simulink model "Communication_Testing"  (R2024a)
settings: Solver=FixedStepAuto  StartTime=0.0  StopTime=100  RelTol=1e-3  EnableMultiTasking=on
undefined symbols (not defined in the file or in its folder): CAN, FD
libraries: stmutilitieslib x29, simulink x25, stm32blockslib x11, canfdmsglib x7, stm32h7xxblockslib x3, dspstat3 x3, slpidlib x2
(part 1 of 2)
settings Model: STM32="{\"FDCANWrite\":[{\"ID\":\"Communication_Testing:678\"},{\"ID\":\"Communication_Testing:677\"},{\"ID\":\"Communication_Testing:1794\"},{\"ID\":\"Communication_Testing:617\"},{\"ID\":\"Communication_Testing:630\"},{\"ID\":\"Communication_Testing:2155\"},{\"ID\":\"Communication_Testing:2156\"}],\"HardwareInterrupt\":[{\"ID\":\"Communication_Testing:1261\"},{\"ID\":\"Communication_Testing:278\"}],\"FDCANRead\":{\"ID\":\"Communication_Testing:282\"},\"AnalogInputForH7\":{\"ID\":\"Communication_Testing:1796\"}}"  Creator=ezeki  LastModifiedBy=ezeki
settings SolverCC: PositivePriorityOrder=on  AutoInsertRateTranBlk=on
settings OptimizationCC: DefaultParameterBehavior=Inlined  EnhancedBackFolding=on  PassReuseOutputArgsAs=Individual arguments  ZeroExternalMemoryAtStartup=off  ZeroInternalMemoryAtStartup=off  MaxStackSize=512  OptimizeBlockOrder=speed  DifferentSizesBufferReuse=on  OptimizationCustomize=off  EfficientTunableParamExpr=on
settings DebuggingCC: ParameterTunabilityLossMsg=error
settings HardwareCC: ProdBitPerPointer=32  ProdBitPerSizeT=32  ProdBitPerPtrDiffT=32  ProdLargestAtomicInteger=Long  ProdLargestAtomicFloat=Double  ProdWordSize=32  ProdLongLongMode=on  ProdHWDeviceType=ARM Compatible->ARM Cortex-M
settings SFSimCC: MATLABDynamicMemAlloc=off
settings RTWCC: Description=Embedded Coder  SystemTargetFile=ert.tlc  HardwareBoard=STM32H7xx Based (Single-core)  TLCOptions="-aInlineSetEventsForThisBaseRateFcn=TLC_FALSE -aSuppressMultiTaskScheduler=TLC_FALSE  -aRateBasedStepFcn=0"  TemplateMakefile=ert_default_tmf  Toolchain=GNU Tools for ARM Embedded Processors  BuildConfiguration=Faster Runs
settings CodeAppCC: ForceParamTrailComments=on  IgnoreCustomStorageClasses=off  OperatorAnnotations=on  SimulinkDataObjDesc=on  SFDataObjDesc=on  InsertBlockDesc=on
settings ERTTargetCC: TargetLangStandard=C99 (ISO)  CodeReplacementLibrary=ARM Cortex-M  ExtModeTransport=3  ExtModeStaticAlloc=on  ExtModeStaticAllocSize=2048  ExtModeMexFile=ext_xcp  ExtModeIntrfLevel=Level2 - Open

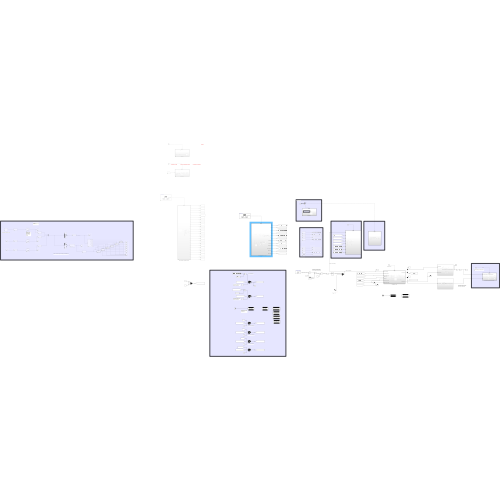
[thumbnail: Simulink's stored preview of the top-level diagram]
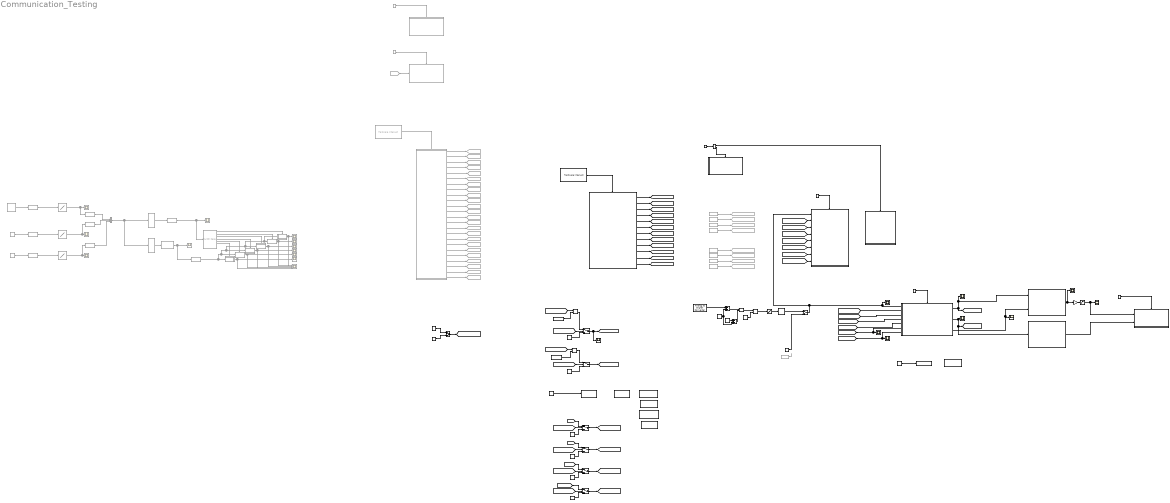
== system Communication_Testing ==
  note: Output to Control Model
  note: Output to CAN for visibility
  note: This invert is done as the right motor spins clockwise. compared to the left motor which spins anticlockwise.
  note: Pot turned down all the way wasnt quite showing 0, this offset was added to ensure 0 throttle could be acheived.
  note: maps 0-3.3V to 0 - 65,536
  note: Traction Control
  note: For testing purposes only
  note: CAN 2 Receive Data From Inverters
  note: Forwarding Messages From the Inverters to Data Logger
  note: This was made for testing the unmultiplexing of Inverter Messages
  note: Inverter Can Setup
  note: A look up table of CAN ID's which are used to request cyclic transmission of data from the inverters
  note: Counter Selects which ID to send
  note: Byte 0 tells the inverters you are setting up cyclic messaging.
  note: CAN 1 information from pedal box and dash.
  note: Set to 500 Hz call
  note: This Constant Can be changed to varible at a latter date for data playback/simulation
  note: Less then 90 enables regen
  note: Greater then 5 enables regen
  note: Greater then 5 enables regen
  note: Converts RPM to Rad/s
  note: This Constant Can be changed to varible at a latter date for data playback/simulation
  note: Example On How to send Messages to Inverters
  note: PID Loop runs allot faster to minimise overshoot. Messages are sent at a slower rate.
  note: Handy to test Can outputs. A constant can be put in to test transmission
  1-D Lookup Table : Lookup_n-D  Commented=on  NumberOfTableDimensions=1  BreakpointsForDimension1=[0 1 2 3 4 5]  Table=[235 74 168 73 95 138]  InterpMethod=Nearest  InternalRulePriority=Speed  RndMeth=Simplest
  1-D Lookup Table1 : Lookup_n-D  Commented=on  NumberOfTableDimensions=1  BreakpointsForDimension1=[0 1 2 3 4 5]  Table=[25 200 25 200 50 50]  InterpMethod=Nearest  InternalRulePriority=Speed  RndMeth=Simplest
  1-D Lookup Table2 : Lookup_n-D  Commented=on  NumberOfTableDimensions=1  BreakpointsForDimension1=[0 1 2 3 4 5]  Table=[25 200 25 200 50 50]  InterpMethod=Nearest  InternalRulePriority=Speed  RndMeth=Simplest
  10 HZ Send : Subsystem  Commented=on  TreatAsAtomicUnit=on
  10 HZ Send1 : Subsystem  TreatAsAtomicUnit=on
  50 HZ Send Torque Requests to Inverters1 : Subsystem  TreatAsAtomicUnit=on
  50 HZ Send1 : Subsystem  Commented=on  TreatAsAtomicUnit=on
  Add : Sum
  Add1 : Sum
  Analog to Digital Converter : stm32h7xxblockslib/Analog to Digital Converter  ADCModule=ADC1  ConversionGroup=Regular  TriggerMode=Trigger and read  NumberOfConversions=1  EnableBufferConv=off  BufferLength=1  OutputStatus=off  SampleTime=-1  EnableSimPort=off  hoistedMaskSrc=ECSoC/ECSimCodegen/Analog to Digital Converter
  Byte Unpack1 : stmutilitieslib/Byte Unpack  Commented=on  dimensions={[1]}  datatypes={'uint16'}  byteAlign=1  blockPlatform=stm32f4discovery
  Constant{,1..3,5..6,10} (7 alike) : Constant  Commented=on  Value=0
  Constant11 : Constant  Commented=on  Value=25000
  Constant12 : Constant  Value=100
  Constant13 : Constant  Value=10000
  Constant14 : Constant  Value=100
  Constant15 : Constant  Value=100
  Constant16 : Constant  Value=0.10472
  Constant17 : Constant  Value=0.10472
  Constant18 : Constant  Value=50
  Constant19 : Constant  Value=85
  Constant20 : Constant  Value=50
  Constant21 : Constant  Value=20
  Constant22 : Constant
  Constant23 : Constant  Value=0
  Constant24 : Constant  Value=580
  Constant4 : Constant  Commented=on
  Constant7 : Constant  Commented=on
  Constant8 : Constant  Value=-100
  Constant9 : Constant  Value=65535
  Counter Limited : simulink/Sources/Counter Limited  Commented=on  uplimit=5  tsamp=0.1
  Counter Limited1 : simulink/Sources/Counter Limited  uplimit=100  tsamp=1
  Data Store Memory : DataStoreMemory  DataStoreName=Battery_Voltage  WriteAfterWriteMsg=warning  ShowAdditionalParam=off
  Data Store Memory1 : DataStoreMemory  DataStoreName=Right_Sim_Discharge_Current  WriteAfterWriteMsg=warning  ShowAdditionalParam=off
  Data Store Memory2 : DataStoreMemory  DataStoreName=Right_Sim_Regen_Current  WriteAfterWriteMsg=warning  ShowAdditionalParam=off
  Data Store Memory3 : DataStoreMemory  DataStoreName=Left_Sim_Discharge_Current  WriteAfterWriteMsg=warning  ShowAdditionalParam=off
  Data Store Memory4 : DataStoreMemory  DataStoreName=Left_Sim_Regen_Current  WriteAfterWriteMsg=warning  ShowAdditionalParam=off
  Data Store Memory5 : DataStoreMemory  DataStoreName=Global_Power_Limit  WriteAfterWriteMsg=warning  ShowAdditionalParam=off
  Data Store Write1 : DataStoreWrite  DataStoreName=Global_Power_Limit  IndexOptions=Index vector (dialog)  Indices=1  OutputSizes=1
  Data Store Write2 : DataStoreWrite  DataStoreName=Battery_Voltage  IndexOptions=Index vector (dialog)  Indices=1  OutputSizes=1
  Data Type Conversion : DataTypeConversion  Commented=on  OutDataTypeStr=uint16  SaturateOnIntegerOverflow=off  RndMeth=Floor
  Data Type Conversion{1,5,7,16} (4 alike) : DataTypeConversion  Commented=on  OutDataTypeStr=double  SaturateOnIntegerOverflow=off  RndMeth=Floor
  Data Type Conversion2 : DataTypeConversion  Commented=on  OutDataTypeStr=uint8  SaturateOnIntegerOverflow=off  RndMeth=Floor
  Data Type Conversion4 : DataTypeConversion  Commented=on  OutDataTypeStr=uint8  SaturateOnIntegerOverflow=off  RndMeth=Floor
  Data Type Conversion6 : DataTypeConversion  Commented=on  OutDataTypeStr=uint8  SaturateOnIntegerOverflow=off  RndMeth=Floor
  Divide : Product  Inputs=*/
  From : From  Commented=on  GotoTag=WSFR
  From File : FromFile  Commented=on  FileName=Pot_input.mat  SampleTime=0
  Function-Call Generator : simulink/Ports & Subsystems/Function-Call Generator  Commented=on  sample_time=0.1  numberOfIterations=1  DisallowWideOutput=off
  Function-Call Generator1 : simulink/Ports & Subsystems/Function-Call Generator  Commented=on  sample_time=0.02  numberOfIterations=1  DisallowWideOutput=off
  Function-Call Generator2 : simulink/Ports & Subsystems/Function-Call Generator  sample_time=0.01  numberOfIterations=1  DisallowWideOutput=off
  Function-Call Generator3 : simulink/Ports & Subsystems/Function-Call Generator  sample_time=0.002  numberOfIterations=1  DisallowWideOutput=off
  Function-Call Generator4 : simulink/Ports & Subsystems/Function-Call Generator  sample_time=0.2  numberOfIterations=1  DisallowWideOutput=off
  Function-Call Generator5 : simulink/Ports & Subsystems/Function-Call Generator  sample_time=0.02  numberOfIterations=1  DisallowWideOutput=off
  Function-Call Split : FunctionCallSplit  IconShape=distinctive  NumOutputPorts=2  OutputPortLayout=default
  Function-Call Subsystem : Subsystem  TreatAsAtomicUnit=on
  Function-Call Subsystem2 : Subsystem  Commented=on  TreatAsAtomicUnit=on
  Gain1 : Gain  Gain=-1
  Goto36 : Goto  Commented=on  GotoTag=CAN_LEFT_Inverter_Bus_Voltage
  Goto37 : Goto  Commented=on  GotoTag=CAN_LEFT_Inverter_Motor_Current
  Goto38 : Goto  Commented=on  GotoTag=CAN_LEFT_Inverter_Motor_Speed
  Goto39 : Goto  Commented=on  GotoTag=CAN_RIGHT_Inverter_Motor_Speed
  Goto40 : Goto  Commented=on  GotoTag=Start_Button
  Goto41 : Goto  Commented=on  GotoTag=CAN_LEFT_Inverter_Motor_Voltage
  Goto42 : Goto  Commented=on  GotoTag=CAN_RIGHT_Inverter_Bus_Voltage
  Goto43 : Goto  Commented=on  GotoTag=SCin
  Goto44 : Goto  Commented=on  GotoTag=SoftwareBSPD
  Goto45 : Goto  Commented=on  GotoTag=CAN_RIGHT_Inverter_Motor_Current
  Goto46 : Goto  Commented=on  GotoTag=SoftwareError
  Goto47 : Goto  Commented=on  GotoTag=CAN_RIGHT_Inverter_Motor_Voltage
  Goto48 : Goto  Commented=on  GotoTag=BSEMatch
  Goto49 : Goto  Commented=on  GotoTag=APPS_Percent
  Goto50 : Goto  Commented=on  GotoTag=Brake_Percent
  Goto51 : Goto  Commented=on  GotoTag=SteeringPercent
  Goto52 : Goto  Commented=on  GotoTag=WSFL
  Goto53 : Goto  Commented=on  GotoTag=WSFR
  Goto54 : Goto  Commented=on  GotoTag=BMS_Current
  Goto55 : Goto  Commented=on  GotoTag=BMS_Voltage
  Goto56 : Goto  Commented=on  GotoTag=SCEstop
  Goto57 : Goto  Commented=on  GotoTag=BMS_SOC
  Goto58 : Goto  Commented=on  GotoTag=BMS_Temprature
  Goto59 : Goto  Commented=on  GotoTag=BMS_Max_CellTemp
  Goto60 : Goto  Commented=on  GotoTag=BMS_Min_CellTemp
  Goto61 : Goto  Commented=on  GotoTag=SCis
  Goto62 : Goto  Commented=on  GotoTag=SCBOTS
  Goto63 : Goto  Commented=on  GotoTag=APPSFail
  Goto64 : Goto  Commented=on  GotoTag=BSEFail
  Goto65 : Goto  Commented=on  GotoTag=SteeringFail
  Goto66 : Goto  Commented=on  GotoTag=APPSMatch
  Goto67 : Goto  Commented=on  GotoTag=BrakesON
  Hardware Interrupt1 : stm32h7xxblockslib/Hardware Interrupt  ISRGroup=Controller Area Network Flexible Data-Rate (FDCAN)  ISRName=FDCAN2_IT0_IRQHandler  ISRNumber=35  EventsList={ 'off', 'FDCAN2 HPME', '1'; 'off', 'FDCAN2 DRXE', '2'; 'on', 'FDCAN2 RF0NE', '3'; 'off', 'FDCAN2 RF0F', '4'; 'off', 'FDCAN2 RF0L', '5'; 'off', 'FDCAN2 RF0W', '6'; 'off', 'FDCAN2 RF1NE', '7'; 'off', 'FDCAN2 RF1F', '8'; 'off', 'FDCAN2 RF1L', '9'; 'off', 'FDCAN2 RF1W', '10'; 'off', 'FDCAN2 TC', '11'; 'off', 'FDCAN2 TCF', '12'; 'off', 'FDCAN2 TFE', '13'; 'off', 'FDCAN2 TEFN', '14'; 'off', 'FDCAN2 TEFL', '15'; 'off', 'FDCAN2 TEFF', '16'; 'off', 'FDCAN2 TEFW', '17'; 'off', 'FDCAN2 TSW', '18'; 'off', 'FDCAN2 MRAF', '19'; 'off', 'FDCAN2 TOO', '20'; 'off', 'FDCAN2 ELO', '21'; 'off', 'FDCAN2 EP', '22'; 'off', 'FDCAN2 EW', '23'; 'off', 'FDCAN2 BO', '24'; 'off', 'FDCAN2 WDI', '25'; 'off', 'FDCAN2 PEA', '26'; 'off', 'FDCAN2 PED', '27'; 'off', 'FDCAN2 ARA', '28'; 'off', 'Custom event', '29' }  SelectedEvents={'FDCAN2 RF0NE'}  TaskPriority=29  DisablePreemption=off  ClearInterruptFlagsAtEndOfEvent=off  InterruptDefinitionFile=$(TARGET_ROOT)/registry/interrupts/STM32F4xxBased_interrupts.xml  HardwareBoard=STM32H7xx Based  EnableSimPort=off
  Hardware Interrupt2 : stm32h7xxblockslib/Hardware Interrupt  Commented=on  ISRGroup=Controller Area Network Flexible Data-Rate (FDCAN)  ISRName=FDCAN1_IT0_IRQHandler  ISRNumber=34  EventsList={ 'off', 'FDCAN1 HPME', '1'; 'off', 'FDCAN1 DRXE', '2'; 'on', 'FDCAN1 RF0NE', '3'; 'off', 'FDCAN1 RF0F', '4'; 'off', 'FDCAN1 RF0L', '5'; 'off', 'FDCAN1 RF0W', '6'; 'off', 'FDCAN1 RF1NE', '7'; 'off', 'FDCAN1 RF1F', '8'; 'off', 'FDCAN1 RF1L', '9'; 'off', 'FDCAN1 RF1W', '10'; 'off', 'FDCAN1 TC', '11'; 'off', 'FDCAN1 TCF', '12'; 'off', 'FDCAN1 TFE', '13'; 'off', 'FDCAN1 TEFN', '14'; 'off', 'FDCAN1 TEFL', '15'; 'off', 'FDCAN1 TEFF', '16'; 'off', 'FDCAN1 TEFW', '17'; 'off', 'FDCAN1 TSW', '18'; 'off', 'FDCAN1 MRAF', '19'; 'off', 'FDCAN1 TOO', '20'; 'off', 'FDCAN1 ELO', '21'; 'off', 'FDCAN1 EP', '22'; 'off', 'FDCAN1 EW', '23'; 'off', 'FDCAN1 BO', '24'; 'off', 'FDCAN1 WDI', '25'; 'off', 'FDCAN1 PEA', '26'; 'off', 'FDCAN1 PED', '27'; 'off', 'FDCAN1 ARA', '28'; 'off', 'Custom event', '29' }  SelectedEvents={'FDCAN1 RF0NE'}  TaskPriority=30  DisablePreemption=off  ClearInterruptFlagsAtEndOfEvent=off  InterruptDefinitionFile=$(TARGET_ROOT)/registry/interrupts/STM32F4xxBased_interrupts.xml  HardwareBoard=STM32H7xx Based  EnableSimPort=off
  If Action Subsystem2 : Subsystem  Commented=on  TreatAsAtomicUnit=on
  If Action Subsystem3 : Subsystem  Commented=on  TreatAsAtomicUnit=on
  If Action Subsystem4 : Subsystem  Commented=on  TreatAsAtomicUnit=on
  If Action Subsystem5 : Subsystem  Commented=on  TreatAsAtomicUnit=on
  If Action Subsystem6 : Subsystem  Commented=on  TreatAsAtomicUnit=on
  If Action Subsystem7 : Subsystem  Commented=on  TreatAsAtomicUnit=on
  Manual Switch : ManualSwitch  CurrentSetting=0
  Manual Switch1 : ManualSwitch
  Moving Average : dspstat3/Moving Average  Method=Sliding window  ForgettingFactorPort=off  SpecifyWindowLength=on  WindowLength=10  OverlapLength=9  AllowArbitraryInputLength=off  ForgettingFactor=0.9  SimulateUsing=Interpreted execution
  Product : Product
  Product1 : Product
  Product2 : Product
  Saturation : Saturate  UpperLimit=100  LowerLimit=0
  Saturation1 : Saturate  UpperLimit=0  LowerLimit=-inf
  Scope{,1..10} (11 alike) : Scope  Commented=on
  Scope11 : Scope  Commented=on  NumInputPorts=6
  Scope{12..20} (9 alike) : Scope
  Selector1 : Selector  Commented=on  InputPortWidth=3  IndexOptions=Index vector (dialog)  Indices=[1 ]  OutputSizes=1
  Selector2 : Selector  Commented=on  InputPortWidth=3  IndexOptions=Index vector (dialog)  Indices=[2 3 ]  OutputSizes=1
  Subsystem1 : Subsystem
  Subsystem2 : Subsystem
  Switch Case1 : SwitchCase  Commented=on  CaseConditions={235, 74, 168, 73, 95, 138}
  Switch{1..2,10,13..15} (6 alike) : Switch  Criteria=u2 > Threshold  Threshold=0.5  SaturateOnIntegerOverflow=off  InputSameDT=off
  Throttle/Regen Control : Subsystem  TreatAsAtomicUnit=on
  Triggered Subsystem : Subsystem  TreatAsAtomicUnit=on
  Triggered Subsystem3 : Subsystem  TreatAsAtomicUnit=on
  Vector Concatenate : Concatenate  Commented=on  NumInputs=3
  wires:
  Function-Call Generator1/1 -> 50 HZ Send1/Trigger
  Function-Call Generator/1 -> 10 HZ Send/Trigger
  From/1 -> 50 HZ Send1/1(In1)
  Hardware Interrupt1/1 -> Function-Call Subsystem/Trigger
  Function-Call Split/2 -> 10 HZ Send1/Trigger
  1-D Lookup Table1/1 -> Data Type Conversion4/1, Scope1/1
  1-D Lookup Table/1 -> Data Type Conversion2/1, Scope/1
  Constant4/1 -> Data Type Conversion1/1
  Data Type Conversion2/1 -> Vector Concatenate/1
  Counter Limited/1 -> Data Type Conversion16/1
  Data Type Conversion16/1 -> 1-D Lookup Table/1
  Data Type Conversion1/1 -> 1-D Lookup Table1/1
  Data Type Conversion4/1 -> Vector Concatenate/2
  Data Type Conversion5/1 -> 1-D Lookup Table2/1
  Constant7/1 -> Data Type Conversion5/1
  Data Type Conversion6/1 -> Vector Concatenate/3
  1-D Lookup Table2/1 -> Data Type Conversion6/1, Scope3/1
  Function-Call Subsystem/2(Out2) -> [CAN_LEFT_Inverter_IGBT_temp]
  Function-Call Subsystem/1(Out1) -> [CAN_LEFT_Inverter_Bus_Voltage]
  Function-Call Subsystem/3(Out3) -> [CAN_LEFT_Inverter_Motor_Speed]
  Function-Call Subsystem/4(Out4) -> [CAN_LEFT_Inverter_Motor_Temp]
  Function-Call Subsystem/5(Out5) -> [CAN_LEFT_Inverter_Motor_Current]
  Function-Call Subsystem/6(Out6) -> [CAN_LEFT_Inverter_Motor_Voltage]
  Function-Call Subsystem/7(Bus Voltage) -> [CAN_RIGHT_Inverter_Bus_Voltage]
  Function-Call Subsystem/8(IGBT Temp) -> [CAN_RIGHT_Inverter_IGBT_temp]
  Function-Call Subsystem/9(Motor Speed) -> [CAN_RIGHT_Inverter_Motor_Speed]
  Function-Call Subsystem/10(Motor Temprature) -> [CAN_RIGHT_Inverter_Motor_Temp]
  Function-Call Subsystem/11(Motor Current) -> [CAN_RIGHT_Inverter_Motor_Current]
  Function-Call Subsystem/12(Motor Voltage) -> [CAN_RIGHT_Inverter_Motor_Voltage]
  Manual Switch1/1 -> Scope14/1, Throttle/Regen Control/1(Throttle Percentage), Triggered Subsystem/1(In1)
  [CAN_LEFT_Inverter_Motor_Speed] -> Triggered Subsystem/2(In2)
  [CAN_LEFT_Inverter_Motor_Current] -> Triggered Subsystem/3(In3)
  [CAN_LEFT_Inverter_Motor_Voltage] -> Triggered Subsystem/4(In4)
  [CAN_RIGHT_Inverter_Bus_Voltage] -> Triggered Subsystem/5(In5)
  [CAN_RIGHT_Inverter_Motor_Speed] -> Triggered Subsystem/6(In6)
  [CAN_RIGHT_Inverter_Motor_Current] -> Triggered Subsystem/7(In7)
  Product/1 -> Saturation/1  "Percentage"
  Constant/1 -> Goto36/1
  Constant2/1 -> Goto38/1
  Constant5/1 -> Goto41/1
  Constant6/1 -> Goto42/1
  Constant10/1 -> Goto45/1
  Constant11/1 -> Goto47/1
  Constant1/1 -> Goto37/1
  Constant3/1 -> Goto39/1
  ? -> ?
  ? -> ?
  ? -> ?
  ? -> ?
  Function-Call Split/1 -> Triggered Subsystem3/Trigger  "10Hz"
  Function-Call Generator4/1 -> Function-Call Split/1  "10Hz"
  Function-Call Subsystem2/23(Out23) -> Goto59/1
  Function-Call Subsystem2/4(Out4) -> Goto61/1
  Function-Call Subsystem2/22(Out22) -> Goto58/1
  Hardware Interrupt2/1 -> Function-Call Subsystem2/Trigger
  Function-Call Subsystem2/6(Out6) -> Goto63/1
  Function-Call Subsystem2/17(Out17) -> Goto52/1
  Function-Call Subsystem2/24(Out24) -> Goto60/1
  Function-Call Subsystem2/7(Out7) -> Goto64/1
  Function-Call Subsystem2/20(Out20) -> Goto55/1
  Function-Call Subsystem2/13(Out13) -> Goto48/1
  Function-Call Subsystem2/8(Out8) -> Goto65/1
  Function-Call Subsystem2/15(Out15) -> Goto50/1
  Function-Call Subsystem2/14(Out14) -> Goto49/1
  Function-Call Subsystem2/12(Out12) -> Goto46/1
  Function-Call Subsystem2/9(Out9) -> Goto66/1
  Function-Call Subsystem2/19(Out19) -> Goto54/1
  Function-Call Subsystem2/16(Out16) -> Goto51/1
  Function-Call Subsystem2/11(Out11) -> Goto44/1
  Function-Call Subsystem2/18(Out18) -> Goto53/1
  Function-Call Subsystem2/3(Out3) -> Goto56/1
  Function-Call Subsystem2/21(Out21) -> Goto57/1
  Function-Call Subsystem2/5(Out5) -> Goto62/1
  Function-Call Subsystem2/10(Out10) -> Goto67/1
  Function-Call Subsystem2/2(Out2) -> Goto43/1
  Function-Call Subsystem2/1(Out1) -> Goto40/1
  Switch Case1/6 -> If Action Subsystem2/Action
  Switch Case1/1 -> If Action Subsystem7/Action
  Byte Unpack1/1 -> Data Type Conversion/1, Scope8/1
  If Action Subsystem3/1(Out1) -> Scope11/5, Scope9/1
  Vector Concatenate/1 -> Selector2/1, Selector1/1
  If Action Subsystem6/1(Out1) -> Scope11/2, Scope4/1
  Switch Case1/3 -> If Action Subsystem5/Action
  Selector1/1 -> Data Type Conversion7/1  "Byte 0"
  If Action Subsystem7/1(Out1) -> Scope11/1, Scope2/1
  If Action Subsystem5/1(Out1) -> Scope11/3, Scope5/1
  If Action Subsystem2/1(Out1) -> Scope11/6, Scope10/1
  Selector2/1 -> Byte Unpack1/1  "Byte 0"
  If Action Subsystem4/1(Out1) -> Scope11/4, Scope7/1
  Switch Case1/2 -> If Action Subsystem6/Action
  Switch Case1/4 -> If Action Subsystem4/Action
  Switch Case1/5 -> If Action Subsystem3/Action
  Data Type Conversion7/1 -> Scope6/1, Switch Case1/1  "Brakes Percentage"
  Data Type Conversion/1 -> If Action Subsystem7/1(In1), If Action Subsystem6/1(In1), If Action Subsystem5/1(In1), If Action Subsystem4/1(In1), If Action Subsystem3/1(In1), If Action Subsystem2/1(In1)
  Function-Call Generator2/1 -> Triggered Subsystem/Trigger
  Analog to Digital Converter/1 -> Add/1
  Constant8/1 -> Add1/2, Add/2
  Add/1 -> Divide/1
  Add1/1 -> Divide/2
  Constant9/1 -> Add1/1
  Divide/1 -> Product/1  "Normalises 0-1"
  Constant12/1 -> Product/2
  [Right_Motor_Speed_Rads] -> Scope16/1, Throttle/Regen Control/7(Right Motor Speed (rads))
  [Battery_Temprature] -> Throttle/Regen Control/4(Battery Temp)
  [Battery_SOC] -> Throttle/Regen Control/5(Battery SOC)
  [Left_Wheel_Speed_Ms] -> Throttle/Regen Control/3(FL Wheel Speed (m/s)1)
  [Right_Wheel_Speed_Ms] -> Throttle/Regen Control/2(FR Wheel Speed (m/s))
  [Left_Motor_Speed_Rads] -> Scope15/1, Throttle/Regen Control/6(Left Motor Speed (rads))
  Function-Call Generator3/1 -> Throttle/Regen Control/Trigger
  Constant13/1 -> Data Store Write1/1
  Constant20/1 -> Switch10/3
  [Simulation_Enable] -> Switch10/2
  Switch10/1 -> [Right_Wheel_Speed_Ms]
  [CAN_RIGHT_Inverter_Motor_Speed] -> Product2/1
  Product2/1 -> Switch2/1
  Constant15/1 -> Switch2/3
  Constant14/1 -> Switch1/3
  [WSFR] -> Switch10/1
  Switch14/1 -> [Battery_SOC]
  [BMS_SOC] -> Switch14/1
  [Simulation_Enable] -> Switch14/2
  [Simulation_Enable] -> Switch1/2
  [Simulation_Enable] -> Switch15/2
  Constant16/1 -> Product1/2
  Constant21/1 -> Switch15/3
  Switch2/1 -> [Right_Motor_Speed_Rads]
  [Simulation_Enable] -> Switch2/2
  [BMS_Temprature] -> Switch15/1
  Constant17/1 -> Product2/2
  Constant19/1 -> Switch14/3
  Switch1/1 -> Scope17/1, [Left_Motor_Speed_Rads]
  Switch13/1 -> [Left_Wheel_Speed_Ms]
  Constant18/1 -> Switch13/3
  Switch15/1 -> [Battery_Temprature]
  [CAN_LEFT_Inverter_Motor_Speed] -> Product1/1
  [Simulation_Enable] -> Switch13/2
  Product1/1 -> Switch1/1
  [WSFL] -> Switch13/1
  Throttle/Regen Control/2(Out2) -> Subsystem2/1(Torque Request), [LeftMotor_Torque_Request], Scope13/1
  Throttle/Regen Control/1(Torque Request) -> [RightMotor_Torque_Request], Subsystem1/1(Torque Request), Scope12/1
  Function-Call Generator5/1 -> 50 HZ Send Torque Requests to Inverters1/Trigger  "50Hz"
  Constant23/1 -> Manual Switch/2  "Simulate"
  Manual Switch/1 -> [Simulation_Enable]
  Constant22/1 -> Manual Switch/1  "Code Gen"
  Constant24/1 -> Data Store Write2/1
  Subsystem1/1(Over Current Protected Torque Request to Inverters) -> Scope19/1, Gain1/1
  Subsystem2/1(Over Current Protected Torque Request to Inverters) -> 50 HZ Send Torque Requests to Inverters1/2(In1)
  Gain1/1 -> Saturation1/1
  Saturation/1 -> Moving Average/1
  From File/1 -> ?
  Moving Average/1 -> Manual Switch1/1  "Noise averaged Percentage"
  Saturation1/1 -> Scope18/1, 50 HZ Send Torque Requests to Inverters1/1(Over Current Protected Torque Request to Inverters)
  Throttle/Regen Control/3(Current Request) -> Scope20/1, Subsystem1/2(Current Request)
  Counter Limited1/1 -> Manual Switch1/2
  [CAN_RIGHT_Inverter_Motor_Voltage] -> Triggered Subsystem/8(In8)

== system Communication_Testing/10 HZ Send ==
  function : TriggerPort  TriggerType=function-call  VariantControl=(inherit)
  Constant : Constant
  Data Type Conversion : DataTypeConversion  OutDataTypeStr=uint8  SaturateOnIntegerOverflow=off  RndMeth=Floor
  FDCAN Write1 : stm32blockslib/FDCAN Write  FDCANModule=FDCAN1  BlockMode=Transmit  OperationReadMode=Data  OperationWriteMode=Data  ReadSource=FIFO 0  BufferNumber=0  OutputTypeReadMode=Unpacked  DataFormatWriteMode=Raw data  CANFrameType=CAN  IdentifierTypeVia=Dialog  IdentifierType=Standard (11-bit identifier)  IdentifierVia=Dialog  Identifier=1200  DataLengthVia=Dialog  DataLength=1  OutputIdType=off  IsBitRateSwitchingEnabled=off  TransmitRemoteFrame=off  OutputFrameType=off  OutputBRS=off  OutputRemoteFrame=off  OutputTxFifoLevel=off  OutputRxFifoLevel=off  OutputStatus=off  Timeout=2  SampleTime=-1
      settings: LibrarySourceBlock=stm32l5xxblockslib/FDCAN Write
  wires:
  Constant/1 -> Data Type Conversion/1
  Data Type Conversion/1 -> FDCAN Write1/1

== system Communication_Testing/10 HZ Send1 ==
  note: Messages to the Inverters are only sent twice at startup. This is total of 12 messages.
  function : TriggerPort  TriggerType=function-call  VariantControl=(inherit)
  Constant : Constant
  Constant1 : Constant  Value=0
  Constant2 : Constant
  Constant3 : Constant  Value=12
  Enabled Subsystem : Subsystem  TreatAsAtomicUnit=on
  GreaterThan : RelationalOperator  Operator=>  OutDataTypeStr=boolean  RndMeth=Simplest  InputSameDT=off
  Scope : Scope
  Scope1 : Scope
  Sum : Sum  Inputs=|++
  Switch : Switch  Criteria=u2 > Threshold  SaturateOnIntegerOverflow=off  InputSameDT=off
  Unit Delay : UnitDelay  SampleTime=-1  HasFrameUpgradeWarning=on
  wires:
  Constant/1 -> Sum/2
  Unit Delay/1 -> Sum/1
  Sum/1 -> GreaterThan/1, Unit Delay/1
  Constant1/1 -> Switch/1
  Constant2/1 -> Switch/3
  Constant3/1 -> GreaterThan/2
  GreaterThan/1 -> Scope1/1, Switch/2
  Switch/1 -> Enabled Subsystem/Enable, Scope/1

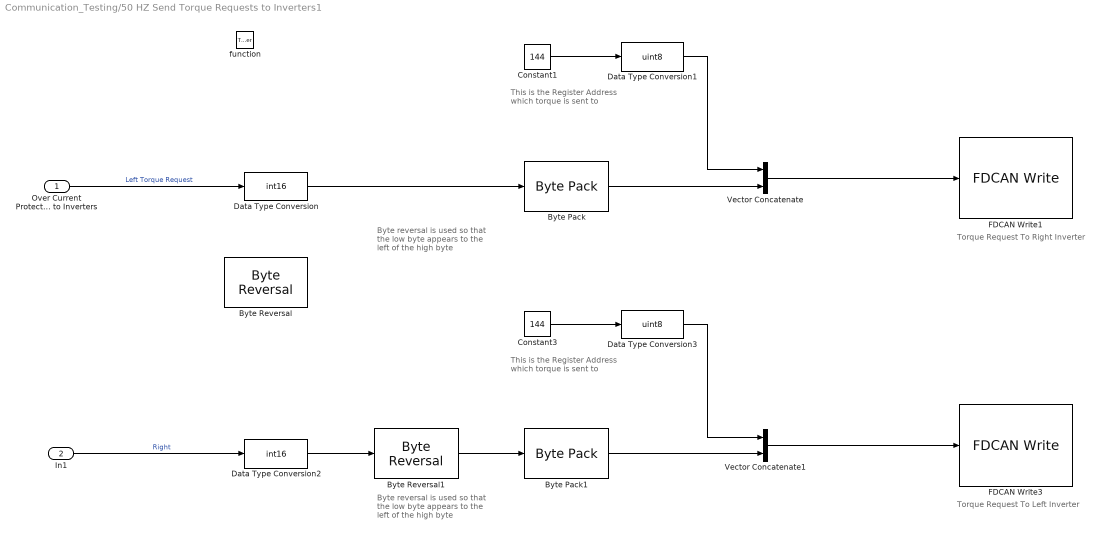
== system Communication_Testing/50 HZ Send Torque Requests to Inverters1 ==
  note: This is the Register Address which torque is sent to
  note: Byte reversal is used so that the low byte appears to the left of the high byte
  note: This is the Register Address which torque is sent to
  note: Byte reversal is used so that the low byte appears to the left of the high byte
  note: Torque Request To Right Inverter
  note: Torque Request To Left Inverter
  Over Current Protected Torque Request to Inverters : Inport
  In1 : Inport  Port=2
  function : TriggerPort  TriggerType=function-call  VariantControl=(inherit)
  Byte Pack : stmutilitieslib/Byte Pack  datatypes={'int16'}  byteAlign=1  blockPlatform=stm32f4discovery
  Byte Pack1 : stmutilitieslib/Byte Pack  datatypes={'int16'}  byteAlign=1  blockPlatform=stm32f4discovery
  Byte Reversal : stmutilitieslib/Byte Reversal  numInp=1  blockPlatform=stm32f4discovery
  Byte Reversal1 : stmutilitieslib/Byte Reversal  numInp=1  blockPlatform=stm32f4discovery
  Constant1 : Constant  Value=144
  Constant3 : Constant  Value=144
  Data Type Conversion : DataTypeConversion  OutDataTypeStr=int16  SaturateOnIntegerOverflow=off  RndMeth=Floor
  Data Type Conversion1 : DataTypeConversion  OutDataTypeStr=uint8  SaturateOnIntegerOverflow=off  RndMeth=Floor
  Data Type Conversion2 : DataTypeConversion  OutDataTypeStr=int16  SaturateOnIntegerOverflow=off  RndMeth=Floor
  Data Type Conversion3 : DataTypeConversion  OutDataTypeStr=uint8  SaturateOnIntegerOverflow=off  RndMeth=Floor
  FDCAN Write1 : stm32blockslib/FDCAN Write  FDCANModule=FDCAN2  BlockMode=Transmit  OperationReadMode=Data  OperationWriteMode=Data  ReadSource=FIFO 0  BufferNumber=0  OutputTypeReadMode=Unpacked  DataFormatWriteMode=Raw data  CANFrameType=CAN  IdentifierTypeVia=Dialog  IdentifierType=Standard (11-bit identifier)  IdentifierVia=Dialog  Identifier=529  DataLengthVia=Dialog  DataLength=3  OutputIdType=off  IsBitRateSwitchingEnabled=off  TransmitRemoteFrame=off  OutputFrameType=off  OutputBRS=off  OutputRemoteFrame=off  OutputTxFifoLevel=off  OutputRxFifoLevel=off  OutputStatus=off  Timeout=1  SampleTime=-1
      settings: LibrarySourceBlock=stm32l5xxblockslib/FDCAN Write
  FDCAN Write3 : stm32blockslib/FDCAN Write  FDCANModule=FDCAN2  BlockMode=Transmit  OperationReadMode=Data  OperationWriteMode=Data  ReadSource=FIFO 0  BufferNumber=0  OutputTypeReadMode=Unpacked  DataFormatWriteMode=Raw data  CANFrameType=CAN  IdentifierTypeVia=Dialog  IdentifierType=Standard (11-bit identifier)  IdentifierVia=Dialog  Identifier=528  DataLengthVia=Dialog  DataLength=3  OutputIdType=off  IsBitRateSwitchingEnabled=off  TransmitRemoteFrame=off  OutputFrameType=off  OutputBRS=off  OutputRemoteFrame=off  OutputTxFifoLevel=off  OutputRxFifoLevel=off  OutputStatus=off  Timeout=1  SampleTime=-1
      settings: LibrarySourceBlock=stm32l5xxblockslib/FDCAN Write
  Vector Concatenate : Concatenate
  Vector Concatenate1 : Concatenate
  wires:
  Over Current Protected Torque Request to Inverters/1 -> Data Type Conversion/1  "Left Torque Request"
  Byte Pack/1 -> Vector Concatenate/2
  Data Type Conversion/1 -> Byte Pack/1
  Vector Concatenate/1 -> FDCAN Write1/1
  Constant1/1 -> Data Type Conversion1/1
  Data Type Conversion1/1 -> Vector Concatenate/1
  Vector Concatenate1/1 -> FDCAN Write3/1
  Byte Pack1/1 -> Vector Concatenate1/2
  In1/1 -> Data Type Conversion2/1  "Right"
  Data Type Conversion3/1 -> Vector Concatenate1/1
  Data Type Conversion2/1 -> Byte Reversal1/1
  Constant3/1 -> Data Type Conversion3/1
  Byte Reversal1/1 -> Byte Pack1/1

== system Communication_Testing/50 HZ Send1 ==
  note: Byte reversal is used so that the low byte appears to the left of the high byte
  In1 : Inport
  function : TriggerPort  TriggerType=function-call  VariantControl=(inherit)
  Add : Sum
  Byte Pack : stmutilitieslib/Byte Pack  datatypes={'uint16'}  byteAlign=1  blockPlatform=stm32f4discovery
  Byte Reversal : stmutilitieslib/Byte Reversal  numInp=1  blockPlatform=stm32f4discovery
  Constant : Constant  Value=1000
  Data Type Conversion : DataTypeConversion  OutDataTypeStr=uint16  SaturateOnIntegerOverflow=off  RndMeth=Floor
  FDCAN Write3 : stm32blockslib/FDCAN Write  FDCANModule=FDCAN1  BlockMode=Transmit  OperationReadMode=Data  OperationWriteMode=Data  ReadSource=FIFO 0  BufferNumber=0  OutputTypeReadMode=Unpacked  DataFormatWriteMode=Raw data  CANFrameType=CAN  IdentifierTypeVia=Dialog  IdentifierType=Standard (11-bit identifier)  IdentifierVia=Dialog  Identifier=1000  DataLengthVia=Dialog  DataLength=2  OutputIdType=off  IsBitRateSwitchingEnabled=off  TransmitRemoteFrame=off  OutputFrameType=off  OutputBRS=off  OutputRemoteFrame=off  OutputTxFifoLevel=off  OutputRxFifoLevel=off  OutputStatus=off  Timeout=1  SampleTime=-1
      settings: LibrarySourceBlock=stm32l5xxblockslib/FDCAN Write
  wires:
  Add/1 -> Data Type Conversion/1
  In1/1 -> Add/1
  Constant/1 -> Add/2
  Data Type Conversion/1 -> Byte Reversal/1
  Byte Pack/1 -> FDCAN Write3/1
  Byte Reversal/1 -> Byte Pack/1

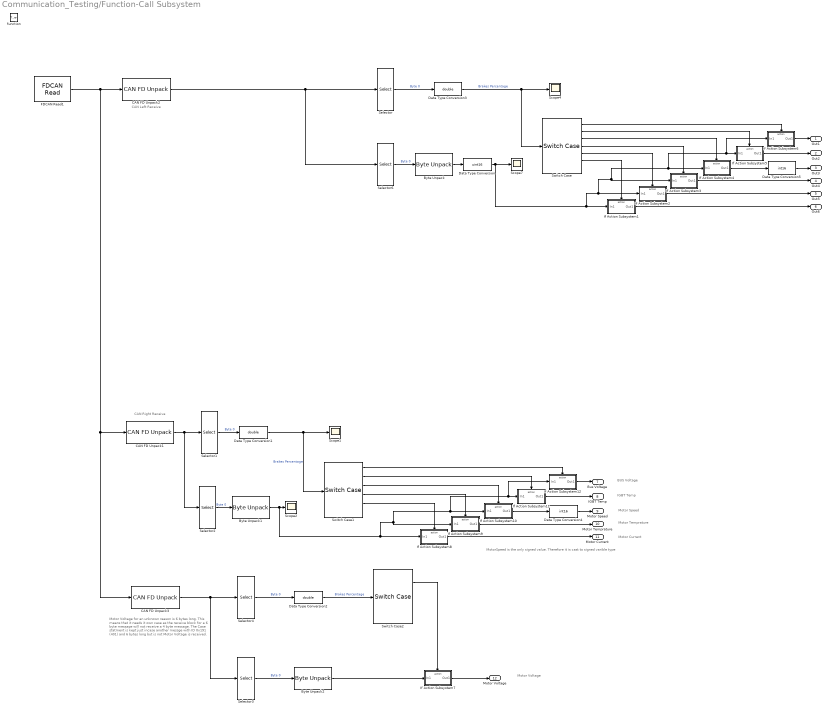
== system Communication_Testing/Function-Call Subsystem ==
  note: BUS Voltage
  note: MotorSpeed is the only signed value. Therefore it is cast to signed varible type
  note: Motor Voltage for an unknown reason is 6 bytes long. This means that it needs it own case as the receive block for a 6 byte message will not receive a 4 byte message. The Case statment is kept just incase another messge with ID 0x191 (401) and 6 bytes long but is not Motor Voltage is received.
  note: CAN Left Receive
  note: CAN Right Receive
  note: IGBT Temp
  note: Motor Speed
  note: Motor Temprature
  note: Motor Current
  note: Motor Voltage
  function : TriggerPort  TriggerType=function-call  VariantControl=(inherit)
  Byte Unpack : stmutilitieslib/Byte Unpack  dimensions={[1]}  datatypes={'uint16'}  byteAlign=1  blockPlatform=stm32f4discovery
  Byte Unpack1 : stmutilitieslib/Byte Unpack  dimensions={[1]}  datatypes={'uint16'}  byteAlign=1  blockPlatform=stm32f4discovery
  Byte Unpack2 : stmutilitieslib/Byte Unpack  dimensions={[1]}  datatypes={'uint16'}  byteAlign=1  blockPlatform=stm32f4discovery
  CAN FD Unpack1 : canfdmsglib/CAN FD Unpack  MsgList=(none)  MsgName=Msg  ProtocolMode=CAN  MsgIDType=Standard (11-bit identifier)  MsgIdentifier=401  MsgLength=4  SignalInfo={}  IDPort=off  TimestampPort=off  ErrorPort=off  RemotePort=off  LengthPort=off  StatusPort=off  BRSPort=off  ESIPort=off  DLCPort=off  ApplyMinMax=off
      settings: LibrarySourceBlock=stmutilitieslib/CAN FD Unpack  DataFormat=raw data
  CAN FD Unpack2 : canfdmsglib/CAN FD Unpack  MsgList=(none)  MsgName=Msg  ProtocolMode=CAN  MsgIDType=Standard (11-bit identifier)  MsgIdentifier=400  MsgLength=3  SignalInfo={}  IDPort=off  TimestampPort=off  ErrorPort=off  RemotePort=off  LengthPort=off  StatusPort=off  BRSPort=off  ESIPort=off  DLCPort=off  ApplyMinMax=off
      settings: LibrarySourceBlock=stmutilitieslib/CAN FD Unpack  DataFormat=raw data
  CAN FD Unpack3 : canfdmsglib/CAN FD Unpack  MsgList=(none)  MsgName=Msg  ProtocolMode=CAN  MsgIDType=Standard (11-bit identifier)  MsgIdentifier=401  MsgLength=6  SignalInfo={}  IDPort=off  TimestampPort=off  ErrorPort=off  RemotePort=off  LengthPort=off  StatusPort=off  BRSPort=off  ESIPort=off  DLCPort=off  ApplyMinMax=off
      settings: LibrarySourceBlock=stmutilitieslib/CAN FD Unpack  DataFormat=raw data
  Data Type Conversion : DataTypeConversion  OutDataTypeStr=uint16  SaturateOnIntegerOverflow=off  RndMeth=Floor
  Data Type Conversion1 : DataTypeConversion  OutDataTypeStr=double  SaturateOnIntegerOverflow=off  RndMeth=Floor
  Data Type Conversion2 : DataTypeConversion  OutDataTypeStr=double  SaturateOnIntegerOverflow=off  RndMeth=Floor
  Data Type Conversion3 : DataTypeConversion  OutDataTypeStr=double  SaturateOnIntegerOverflow=off  RndMeth=Floor
  Data Type Conversion4 : DataTypeConversion  OutDataTypeStr=int16  SaturateOnIntegerOverflow=off  RndMeth=Floor
  Data Type Conversion5 : DataTypeConversion  OutDataTypeStr=int16  SaturateOnIntegerOverflow=off  RndMeth=Floor
  FDCAN Read1 : stm32blockslib/FDCAN Read  FDCANModule=FDCAN2  BlockMode=Receive  OperationReadMode=Data  OperationWriteMode=Data  ReadSource=FIFO 0  BufferNumber=0  OutputTypeReadMode=Packed  DataFormatWriteMode=Raw data  CANFrameType=CAN-FD  IdentifierTypeVia=Dialog  IdentifierType=Standard (11-bit identifier)  IdentifierVia=Inport  Identifier=100  DataLengthVia=Inport  DataLength=64  OutputIdType=off  IsBitRateSwitchingEnabled=off  TransmitRemoteFrame=off  OutputFrameType=off  OutputBRS=off  OutputRemoteFrame=off  OutputTxFifoLevel=off  OutputRxFifoLevel=off  OutputStatus=off  Timeout=0.001  SampleTime=-1
      settings: LibrarySourceBlock=stm32l5xxblockslib/FDCAN Read
  If Action Subsystem1 : Subsystem  TreatAsAtomicUnit=on
  If Action Subsystem10 : Subsystem  TreatAsAtomicUnit=on
  If Action Subsystem11 : Subsystem  TreatAsAtomicUnit=on
  If Action Subsystem12 : Subsystem  TreatAsAtomicUnit=on
  If Action Subsystem2 : Subsystem  TreatAsAtomicUnit=on
  If Action Subsystem3 : Subsystem  TreatAsAtomicUnit=on
  If Action Subsystem4 : Subsystem  TreatAsAtomicUnit=on
  If Action Subsystem5 : Subsystem  TreatAsAtomicUnit=on
  If Action Subsystem6 : Subsystem  TreatAsAtomicUnit=on
  If Action Subsystem7 : Subsystem  TreatAsAtomicUnit=on
  If Action Subsystem8 : Subsystem  TreatAsAtomicUnit=on
  If Action Subsystem9 : Subsystem  TreatAsAtomicUnit=on
  Scope{1..2,4,7} (4 alike) : Scope
  Selector : Selector  InputPortWidth=3  IndexOptions=Index vector (dialog)  Indices=[1 ]  OutputSizes=1
  Selector1 : Selector  InputPortWidth=4  IndexOptions=Index vector (dialog)  Indices=[1 ]  OutputSizes=1
  Selector2 : Selector  InputPortWidth=4  IndexOptions=Index vector (dialog)  Indices=[2 3 ]  OutputSizes=1
  Selector3 : Selector  InputPortWidth=6  IndexOptions=Index vector (dialog)  Indices=[2 3 ]  OutputSizes=1
  Selector4 : Selector  InputPortWidth=6  IndexOptions=Index vector (dialog)  Indices=[1 ]  OutputSizes=1
  Selector6 : Selector  InputPortWidth=3  IndexOptions=Index vector (dialog)  Indices=[2 3 ]  OutputSizes=1
  Switch Case : SwitchCase  CaseConditions={235, 74, 168, 73, 95, 138}
  Switch Case1 : SwitchCase  CaseConditions={235, 74, 168, 73, 95}
  Switch Case2 : SwitchCase  CaseConditions={138}
  Out1 : Outport
  Out2 : Outport  Port=2
  Out3 : Outport  Port=3
  Out4 : Outport  Port=4
  Out5 : Outport  Port=5
  Out6 : Outport  Port=6
  Bus Voltage : Outport  Port=7
  IGBT Temp : Outport  Port=8
  Motor Speed : Outport  Port=9
  Motor Temprature : Outport  Port=10
  Motor Current : Outport  Port=11
  Motor Voltage : Outport  Port=12
  wires:
  FDCAN Read1/1 -> CAN FD Unpack1/1, CAN FD Unpack3/1, CAN FD Unpack2/1
  CAN FD Unpack2/1 -> Selector6/1, Selector/1
  Selector/1 -> Data Type Conversion3/1  "Byte 0"
  Data Type Conversion3/1 -> Scope4/1, Switch Case/1  "Brakes Percentage"
  Byte Unpack/1 -> Data Type Conversion/1
  Selector6/1 -> Byte Unpack/1  "Byte 0"
  Switch Case/6 -> If Action Subsystem1/Action
  If Action Subsystem1/1(Out1) -> Out6/1
  Switch Case/5 -> If Action Subsystem2/Action
  Switch Case/4 -> If Action Subsystem3/Action
  Switch Case/3 -> If Action Subsystem4/Action
  Switch Case/2 -> If Action Subsystem5/Action
  Switch Case/1 -> If Action Subsystem6/Action
  If Action Subsystem6/1(Out1) -> Out1/1
  If Action Subsystem5/1(Out1) -> Out2/1
  If Action Subsystem4/1(Out1) -> Data Type Conversion5/1
  If Action Subsystem2/1(Out1) -> Out5/1
  If Action Subsystem3/1(Out1) -> Out4/1
  Selector2/1 -> Byte Unpack1/1  "Byte 0"
  Byte Unpack1/1 -> If Action Subsystem12/1(In1), If Action Subsystem11/1(In1), If Action Subsystem10/1(In1), If Action Subsystem9/1(In1), If Action Subsystem8/1(In1), Scope2/1
  Data Type Conversion1/1 -> Scope1/1, Switch Case1/1  "Brakes Percentage"
  If Action Subsystem10/1(Out1) -> Data Type Conversion4/1
  Switch Case1/2 -> If Action Subsystem11/Action
  Switch Case1/3 -> If Action Subsystem10/Action
  Selector1/1 -> Data Type Conversion1/1  "Byte 0"
  If Action Subsystem11/1(Out1) -> IGBT Temp/1
  If Action Subsystem9/1(Out1) -> Motor Temprature/1
  If Action Subsystem12/1(Out1) -> Bus Voltage/1
  Switch Case1/5 -> If Action Subsystem8/Action
  Switch Case1/4 -> If Action Subsystem9/Action
  If Action Subsystem8/1(Out1) -> Motor Current/1
  Switch Case1/1 -> If Action Subsystem12/Action
  CAN FD Unpack1/1 -> Selector2/1, Selector1/1
  Data Type Conversion/1 -> If Action Subsystem6/1(In1), If Action Subsystem5/1(In1), If Action Subsystem4/1(In1), If Action Subsystem3/1(In1), If Action Subsystem2/1(In1), If Action Subsystem1/1(In1), Scope7/1
  Selector3/1 -> Byte Unpack2/1  "Byte 0"
  Selector4/1 -> Data Type Conversion2/1  "Byte 0"
  CAN FD Unpack3/1 -> Selector3/1, Selector4/1
  Data Type Conversion2/1 -> Switch Case2/1  "Brakes Percentage"
  Switch Case2/1 -> If Action Subsystem7/Action
  Byte Unpack2/1 -> If Action Subsystem7/1(In1)
  If Action Subsystem7/1(Out1) -> Motor Voltage/1
  Data Type Conversion4/1 -> Motor Speed/1
  Data Type Conversion5/1 -> Out3/1

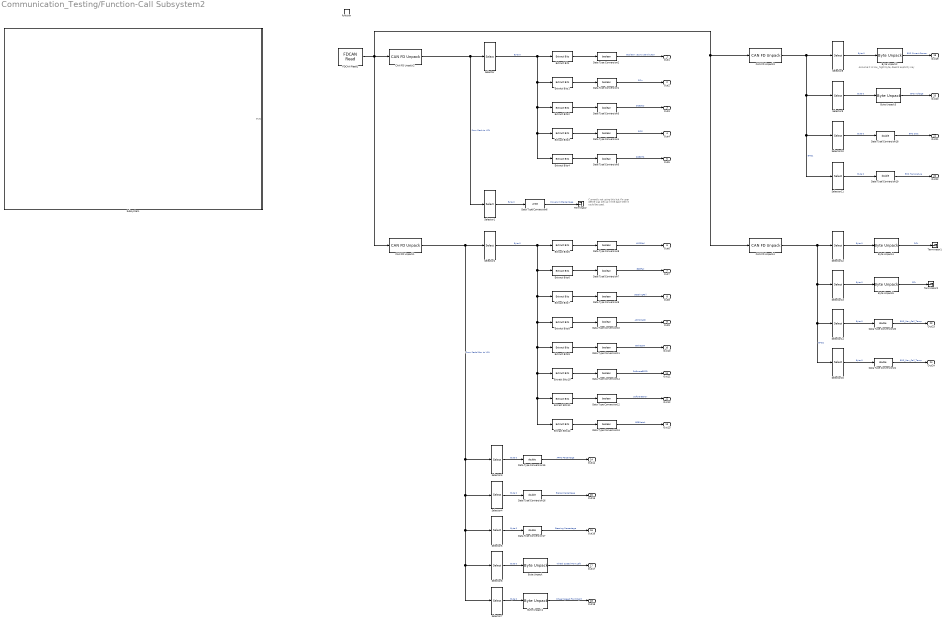
== system Communication_Testing/Function-Call Subsystem2 ==
  note: Assume it is low_hight byte, doesnt explicity say
  note: Currently not using this but if a user define was set up in the dash then it could be used.
  function : TriggerPort  TriggerType=function-call  VariantControl=(inherit)
  Byte Unpack{,1..5} (6 alike) : stmutilitieslib/Byte Unpack  dimensions={[1]}  datatypes={'uint16'}  byteAlign=1  blockPlatform=stm32f4discovery
  CAN FD Unpack1 : canfdmsglib/CAN FD Unpack  MsgList=(none)  MsgName=Msg  ProtocolMode=CAN  MsgIDType=Standard (11-bit identifier)  MsgIdentifier=1  MsgLength=8  SignalInfo={}  IDPort=off  TimestampPort=off  ErrorPort=off  RemotePort=off  LengthPort=off  StatusPort=off  BRSPort=off  ESIPort=off  DLCPort=off  ApplyMinMax=off
      settings: LibrarySourceBlock=stmutilitieslib/CAN FD Unpack  DataFormat=raw data
  CAN FD Unpack2 : canfdmsglib/CAN FD Unpack  MsgList=(none)  MsgName=Msg  ProtocolMode=CAN  MsgIDType=Standard (11-bit identifier)  MsgIdentifier=2  MsgLength=8  SignalInfo={}  IDPort=off  TimestampPort=off  ErrorPort=off  RemotePort=off  LengthPort=off  StatusPort=off  BRSPort=off  ESIPort=off  DLCPort=off  ApplyMinMax=off
      settings: LibrarySourceBlock=stmutilitieslib/CAN FD Unpack  DataFormat=raw data
  CAN FD Unpack3 : canfdmsglib/CAN FD Unpack  MsgList=(none)  MsgName=Msg  ProtocolMode=CAN  MsgIDType=Standard (11-bit identifier)  MsgIdentifier=4  MsgLength=8  SignalInfo={}  IDPort=off  TimestampPort=off  ErrorPort=off  RemotePort=off  LengthPort=off  StatusPort=off  BRSPort=off  ESIPort=off  DLCPort=off  ApplyMinMax=off
      settings: LibrarySourceBlock=stmutilitieslib/CAN FD Unpack  DataFormat=raw data
  CAN FD Unpack4 : canfdmsglib/CAN FD Unpack  MsgList=(none)  MsgName=Msg  ProtocolMode=CAN  MsgIDType=Standard (11-bit identifier)  MsgIdentifier=5  MsgLength=8  SignalInfo={}  IDPort=off  TimestampPort=off  ErrorPort=off  RemotePort=off  LengthPort=off  StatusPort=off  BRSPort=off  ESIPort=off  DLCPort=off  ApplyMinMax=off
      settings: LibrarySourceBlock=stmutilitieslib/CAN FD Unpack  DataFormat=raw data
  Data Type Conversion{1..5,7..14} (13 alike) : DataTypeConversion  OutDataTypeStr=boolean  SaturateOnIntegerOverflow=off  RndMeth=Floor
  Data Type Conversion{15..21} (7 alike) : DataTypeConversion  OutDataTypeStr=double  SaturateOnIntegerOverflow=off  RndMeth=Floor
  Data Type Conversion6 : DataTypeConversion  OutDataTypeStr=uint8  SaturateOnIntegerOverflow=off  RndMeth=Floor
  Extract Bits : simulink/Logic and Bit Operations/Extract Bits  bitsToExtract=Range of bits  numBits=8  bitIdxRange=[0]  outScalingMode=Treat bit field as an integer
  Extract Bits1 : simulink/Logic and Bit Operations/Extract Bits  bitsToExtract=Range of bits  numBits=8  bitIdxRange=[3]  outScalingMode=Treat bit field as an integer
  Extract Bits10 : simulink/Logic and Bit Operations/Extract Bits  bitsToExtract=Range of bits  numBits=8  bitIdxRange=[5]  outScalingMode=Treat bit field as an integer
  Extract Bits11 : simulink/Logic and Bit Operations/Extract Bits  bitsToExtract=Range of bits  numBits=8  bitIdxRange=[6]  outScalingMode=Treat bit field as an integer
  Extract Bits12 : simulink/Logic and Bit Operations/Extract Bits  bitsToExtract=Range of bits  numBits=8  bitIdxRange=[7]  outScalingMode=Treat bit field as an integer
  Extract Bits2 : simulink/Logic and Bit Operations/Extract Bits  bitsToExtract=Range of bits  numBits=8  bitIdxRange=[4]  outScalingMode=Treat bit field as an integer
  Extract Bits3 : simulink/Logic and Bit Operations/Extract Bits  bitsToExtract=Range of bits  numBits=8  bitIdxRange=[5]  outScalingMode=Treat bit field as an integer
  Extract Bits4 : simulink/Logic and Bit Operations/Extract Bits  bitsToExtract=Range of bits  numBits=8  bitIdxRange=[6]  outScalingMode=Treat bit field as an integer
  Extract Bits5 : simulink/Logic and Bit Operations/Extract Bits  bitsToExtract=Range of bits  numBits=8  bitIdxRange=[0]  outScalingMode=Treat bit field as an integer
  Extract Bits6 : simulink/Logic and Bit Operations/Extract Bits  bitsToExtract=Range of bits  numBits=8  bitIdxRange=[1]  outScalingMode=Treat bit field as an integer
  Extract Bits7 : simulink/Logic and Bit Operations/Extract Bits  bitsToExtract=Range of bits  numBits=8  bitIdxRange=[2]  outScalingMode=Treat bit field as an integer
  Extract Bits8 : simulink/Logic and Bit Operations/Extract Bits  bitsToExtract=Range of bits  numBits=8  bitIdxRange=[3]  outScalingMode=Treat bit field as an integer
  Extract Bits9 : simulink/Logic and Bit Operations/Extract Bits  bitsToExtract=Range of bits  numBits=8  bitIdxRange=[4]  outScalingMode=Treat bit field as an integer
  FDCAN Read1 : stm32blockslib/FDCAN Read  FDCANModule=FDCAN1  BlockMode=Receive  OperationReadMode=Data  OperationWriteMode=Data  ReadSource=FIFO 0  BufferNumber=0  OutputTypeReadMode=Packed  DataFormatWriteMode=Raw data  CANFrameType=CAN-FD  IdentifierTypeVia=Dialog  IdentifierType=Standard (11-bit identifier)  IdentifierVia=Inport  Identifier=100  DataLengthVia=Inport  DataLength=64  OutputIdType=off  IsBitRateSwitchingEnabled=off  TransmitRemoteFrame=off  OutputFrameType=off  OutputBRS=off  OutputRemoteFrame=off  OutputTxFifoLevel=off  OutputRxFifoLevel=off  OutputStatus=off  Timeout=0.001  SampleTime=-1
      settings: LibrarySourceBlock=stm32l5xxblockslib/FDCAN Read
  Selector : Selector  InputPortWidth=8  IndexOptions=Index vector (dialog)  Indices=[1 ]  OutputSizes=1
  Selector1 : Selector  InputPortWidth=8  IndexOptions=Index vector (dialog)  Indices=[2 ]  OutputSizes=1
  Selector{10..11,14..15} (4 alike) : Selector  InputPortWidth=8  IndexOptions=Index vector (dialog)  Indices=[5 ]  OutputSizes=1
  Selector12 : Selector  InputPortWidth=8  IndexOptions=Index vector (dialog)  Indices=[1 2 ]  OutputSizes=1
  Selector13 : Selector  InputPortWidth=8  IndexOptions=Index vector (dialog)  Indices=[3 4 ]  OutputSizes=1
  Selector2 : Selector  InputPortWidth=8  IndexOptions=Index vector (dialog)  Indices=[1 ]  OutputSizes=1
  Selector3 : Selector  InputPortWidth=8  IndexOptions=Index vector (dialog)  Indices=[2 ]  OutputSizes=1
  Selector4 : Selector  InputPortWidth=8  IndexOptions=Index vector (dialog)  Indices=[3 ]  OutputSizes=1
  Selector5 : Selector  InputPortWidth=8  IndexOptions=Index vector (dialog)  Indices=[4 ]  OutputSizes=1
  Selector6 : Selector  InputPortWidth=8  IndexOptions=Index vector (dialog)  Indices=[5 6 ]  OutputSizes=1
  Selector7 : Selector  InputPortWidth=8  IndexOptions=Index vector (dialog)  Indices=[7 8 ]  OutputSizes=1
  Selector8 : Selector  InputPortWidth=8  IndexOptions=Index vector (dialog)  Indices=[1 2 ]  OutputSizes=1
  Selector9 : Selector  InputPortWidth=8  IndexOptions=Index vector (dialog)  Indices=[3 4 ]  OutputSizes=1
  Subsystem : Subsystem
      mask Display: image('ALL Can.jpg');
  Terminator : Terminator
  Terminator1 : Terminator
  Terminator2 : Terminator
  Out1 : Outport
  Out2 : Outport  Port=2
  Out3 : Outport  Port=3
  Out4 : Outport  Port=4
  Out5 : Outport  Port=5
  Out6 : Outport  Port=6
  Out7 : Outport  Port=7
  Out8 : Outport  Port=8
  Out9 : Outport  Port=9
  Out10 : Outport  Port=10
  Out11 : Outport  Port=11
  Out12 : Outport  Port=12
  Out13 : Outport  Port=13
  Out14 : Outport  Port=14
  Out15 : Outport  Port=15
  Out16 : Outport  Port=16
  Out17 : Outport  Port=17
  Out18 : Outport  Port=18
  Out19 : Outport  Port=19
  Out20 : Outport  Port=20
  Out21 : Outport  Port=21
  Out22 : Outport  Port=22
  Out23 : Outport  Port=23
  Out24 : Outport  Port=24
  wires:
  CAN FD Unpack2/1 -> Selector1/1, Selector/1  "From Dash to VCU"
  FDCAN Read1/1 -> CAN FD Unpack1/1, CAN FD Unpack4/1, CAN FD Unpack3/1, CAN FD Unpack2/1
  Selector/1 -> Extract Bits4/1, Extract Bits3/1, Extract Bits2/1, Extract Bits1/1, Extract Bits/1  "Byte 0"
  Extract Bits/1 -> Data Type Conversion2/1
  Data Type Conversion2/1 -> Out1/1  "Boolean yes/no start button"
  Extract Bits1/1 -> Data Type Conversion1/1
  Data Type Conversion1/1 -> Out2/1  "SCin"
  Extract Bits2/1 -> Data Type Conversion3/1
  Data Type Conversion3/1 -> Out3/1  "SCEstop"
  Extract Bits3/1 -> Data Type Conversion4/1
  Data Type Conversion4/1 -> Out4/1  "SCIS"
  Extract Bits4/1 -> Data Type Conversion5/1
  Data Type Conversion5/1 -> Out5/1  "SCBOTS"
  Selector1/1 -> Data Type Conversion6/1  "Byte 0"
  Data Type Conversion6/1 -> Terminator/1  "PowerLimitPercentage"
  CAN FD Unpack1/1 -> Selector7/1, Selector6/1, Selector5/1, Selector4/1, Selector3/1, Selector2/1  "From Pedal Box to VCU"
  Data Type Conversion9/1 -> Out8/1  "SteeringFail"
  Extract Bits7/1 -> Data Type Conversion9/1
  Extract Bits6/1 -> Data Type Conversion7/1
  Extract Bits9/1 -> Data Type Conversion11/1
  Extract Bits5/1 -> Data Type Conversion8/1
  Extract Bits8/1 -> Data Type Conversion10/1
  Data Type Conversion7/1 -> Out7/1  "BSEFail"
  Data Type Conversion8/1 -> Out6/1  "APPSFail"
  Data Type Conversion10/1 -> Out9/1  "APPSMatch"
  Data Type Conversion11/1 -> Out10/1  "BrakesON"
  Extract Bits11/1 -> Data Type Conversion12/1
  Extract Bits12/1 -> Data Type Conversion13/1
  Data Type Conversion13/1 -> Out13/1  "BSEMatch"
  Selector2/1 -> Extract Bits12/1, Extract Bits11/1, Extract Bits10/1, Extract Bits9/1, Extract Bits8/1, Extract Bits7/1, Extract Bits6/1, Extract Bits5/1  "Byte 0"
  Data Type Conversion12/1 -> Out12/1  "SoftwareError"
  Data Type Conversion14/1 -> Out11/1  "SoftwareBSPD"
  Extract Bits10/1 -> Data Type Conversion14/1
  Selector3/1 -> Data Type Conversion15/1  "Byte 0"
  Data Type Conversion15/1 -> Out14/1  "APPS Percentage"
  Selector4/1 -> Data Type Conversion16/1  "Byte 0"
  Data Type Conversion16/1 -> Out15/1  "Brakes Percentage"
  Selector5/1 -> Data Type Conversion17/1  "Byte 0"
  Data Type Conversion17/1 -> Out16/1  "Steering Percentage"
  Selector6/1 -> Byte Unpack/1  "Byte 0"
  Byte Unpack/1 -> Out17/1  "Wheel Speed Front Left"
  Selector7/1 -> Byte Unpack1/1  "Byte 0"
  Byte Unpack1/1 -> Out18/1  "Wheel Speed Front Right"
  CAN FD Unpack3/1 -> Selector11/1, Selector10/1, Selector9/1, Selector8/1  "BMS1"
  Selector8/1 -> Byte Unpack2/1  "Byte 0"
  Byte Unpack2/1 -> Out19/1  "BMS Current Sensor"
  Selector9/1 -> Byte Unpack3/1  "Byte 0"
  Byte Unpack3/1 -> Out20/1  "BMS Voltage"
  Selector10/1 -> Data Type Conversion18/1  "Byte 0"
  Data Type Conversion18/1 -> Out21/1  "BMS SOC"
  Selector11/1 -> Data Type Conversion19/1  "Byte 0"
  Data Type Conversion19/1 -> Out22/1  "BMS Temprature"
  CAN FD Unpack4/1 -> Selector15/1, Selector14/1, Selector13/1, Selector12/1  "BMS2"
  Selector12/1 -> Byte Unpack4/1  "Byte 0"
  Byte Unpack4/1 -> Terminator1/1  "DCL"
  Selector13/1 -> Byte Unpack5/1  "Byte 0"
  Byte Unpack5/1 -> Terminator2/1  "CCL"
  Selector14/1 -> Data Type Conversion20/1  "Byte 0"
  Data Type Conversion20/1 -> Out23/1  "BMS_Max_Cell_Temp"
  Selector15/1 -> Data Type Conversion21/1  "Byte 0"
  Data Type Conversion21/1 -> Out24/1  "BMS_Max_Cell_Temp"

== system Communication_Testing/If Action Subsystem2 ==
  In1 : Inport
  Action Port : ActionPort  ActionPortLabel=case [ 138 ]:
  Out1 : Outport
  wires:
  In1/1 -> Out1/1

== system Communication_Testing/If Action Subsystem3 ==
  In1 : Inport
  Action Port : ActionPort  ActionPortLabel=case [ 95 ]:
  Out1 : Outport
  wires:
  In1/1 -> Out1/1

== system Communication_Testing/If Action Subsystem4 ==
  In1 : Inport
  Action Port : ActionPort  ActionPortLabel=case [ 73 ]:
  Out1 : Outport
  wires:
  In1/1 -> Out1/1

== system Communication_Testing/If Action Subsystem5 ==
  In1 : Inport
  Action Port : ActionPort  ActionPortLabel=case [ 168 ]:
  Out1 : Outport
  wires:
  In1/1 -> Out1/1

== system Communication_Testing/If Action Subsystem6 ==
  In1 : Inport
  Action Port : ActionPort  ActionPortLabel=case [ 74 ]:
  Out1 : Outport
  wires:
  In1/1 -> Out1/1
